simulink model "assignmenttest"  (Simulink 7.6)
settings: Solver=FixedStepDiscrete  StartTime=0.0  StopTime=1  FixedStep=1  RelTol=1e-3
settings Model: Creator=c2wt  LastModifiedBy=c2wt
settings DataIOCC: SaveFormat=Structure

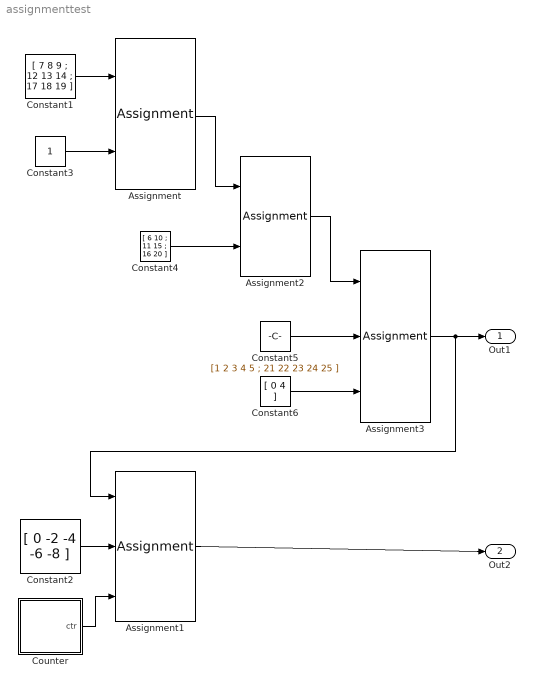
== system assignmenttest ==
  Assignment : Assignment  NumberOfDimensions=2  IndexMode=Zero-based  OutputInitialize=Specify size for each dimension in table  IndexOptions=Starting index (dialog),Starting index (port)  Indices=1,1  OutputSizes=5,5
  Assignment1 : Assignment  NumberOfDimensions=2  IndexMode=Zero-based  IndexOptions=Starting index (port),Assign all  Indices=1,[1 2 4 5 7]  OutputSizes=1,1
  Assignment2 : Assignment  NumberOfDimensions=2  IndexMode=Zero-based  IndexOptions=Starting index (dialog),Index vector (dialog)  Indices=1,[0 4]  OutputSizes=1,1
  Assignment3 : Assignment  NumberOfDimensions=2  IndexMode=Zero-based  IndexOptions=Index vector (port),Assign all  Indices=1,1  OutputSizes=1,1
  Constant1 : Constant  Value=[ 7 8 9 ; 12 13 14 ; 17 18 19 ]
  Constant2 : Constant  Value=[ 0 -2 -4 -6 -8 ]  VectorParams1D=off
  Constant3 : Constant
  Constant4 : Constant  Value=[ 6 10 ; 11 15 ; 16 20 ]
  Constant5 : Constant  Value=[1 2 3 4 5 ; 21 22 23 24 25 ]
  Constant6 : Constant  Value=[ 0 4 ]
  Counter : Stateflow chart  TreatAsAtomicUnit=on
  Out1 : Outport
  Out2 : Outport  Port=2
  wires:
  Assignment1/1 -> Out2/1
  Constant1/1 -> Assignment/1
  Constant3/1 -> Assignment/2
  Assignment/1 -> Assignment2/1
  Constant4/1 -> Assignment2/2
  Assignment2/1 -> Assignment3/1
  Constant5/1 -> Assignment3/2
  Constant6/1 -> Assignment3/3
  Assignment3/1 -> Assignment1/1, Out1/1
  Constant2/1 -> Assignment1/2
  Counter/1(ctr) -> Assignment1/3

== stateflow chart Counter ==
  state s1
  (default) -> s1
  s1 -> s1 [order 1] : [ctr < 4] / ctr = ctr+1;
  s1 -> s1 [order 2] : [ctr >= 4] / ctr = 0;
  data: ctr output double =1
